simulink model "q4"  (R2020b)
settings: Solver=VariableStepAuto  StartTime=0.0  StopTime=10  RelTol=1e-3
values from neighbouring files (symbols this model uses):
  b = 3.5077E-6    [position_data.sldd]
  J = 3.2284E-6    [position_data.sldd]
  ke = 0.0274    [position_data.sldd]
  kt = 0.0274    [position_data.sldd]
  L = 2.75E-6    [position_data.sldd]
  R = 4.0    [position_data.sldd]
settings Model: DataDictionary=position_data.sldd  Creator=Ravi  LastModifiedBy=Ravi

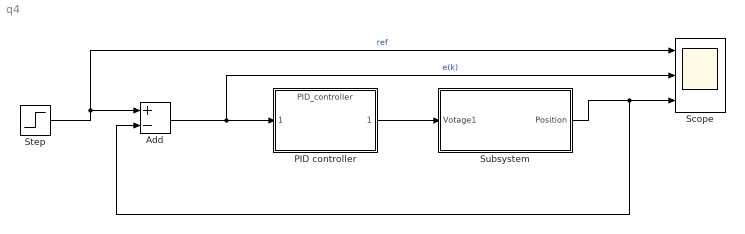
== system q4 ==
  Add : Sum  Inputs=+-
  PID controller : ModelReference  ModelNameDialog=PID_controller  SimulationMode=Normal  ModelReferenceVersion=1.6
  Scope : Scope  NumInputPorts=3
  Step : Step  SampleTime=0
  Subsystem : Subsystem
  wires:
  Add/1 -> Scope/2, PID controller/1  "e(k)"
  Step/1 -> Scope/1, Add/1  "ref"
  PID controller/1 -> Subsystem/1(Votage1)
  Subsystem/1(Position) -> Add/2, Scope/3

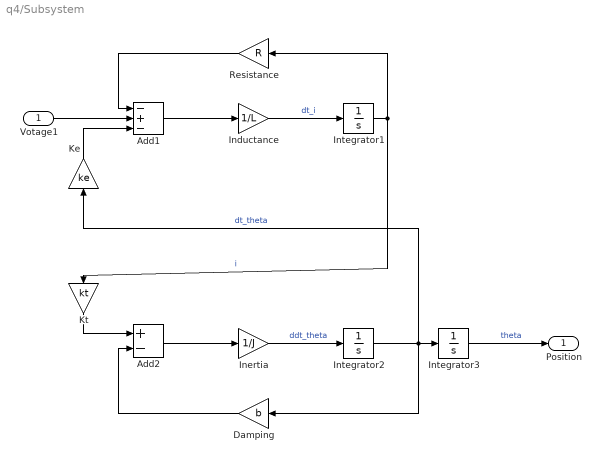
== system q4/Subsystem ==
  Votage1 : Inport
  Add1 : Sum  Inputs=-+-
  Add2 : Sum  Inputs=+-
  Damping : Gain  Gain=b
  Inductance : Gain  Gain=1/L
  Inertia : Gain  Gain=1/J
  Integrator1 : Integrator
  Integrator2 : Integrator
  Integrator3 : Integrator
  Ke : Gain  Gain=ke
  Kt : Gain  Gain=kt
  Resistance : Gain  Gain=R
  Position : Outport
  wires:
  Add2/1 -> Inertia/1
  Add1/1 -> Inductance/1
  Integrator2/1 -> Ke/1, Integrator3/1, Damping/1  "dt_theta"
  Resistance/1 -> Add1/1
  Ke/1 -> Add1/3
  Inertia/1 -> Integrator2/1  "ddt_theta"
  Votage1/1 -> Add1/2
  Inductance/1 -> Integrator1/1  "dt_i"
  Integrator1/1 -> Resistance/1, Kt/1  "i"
  Integrator3/1 -> Position/1  "theta"
  Kt/1 -> Add2/1
  Damping/1 -> Add2/2
